simulink library "MAN_Library"  (R2023a)
settings: Solver=ode45  StartTime=0.0  StopTime=10.0  RelTol=1e-3  EnableMultiTasking=on
undefined symbols (not defined in the file): EventID
libraries: $bdroot x33, simulink_need_slupdate x1
(part 1 of 2)
settings Model: Creator=u23d01  LastModifiedBy=u29w13
settings SolverCC: AlgebraicLoopSolver=TrustRegion
settings DataIOCC: LimitDataPoints=on  SaveFormat=Array  ReturnWorkspaceOutputs=off
settings OptimizationCC: LifeSpan=inf
settings DebuggingCC: UnderspecifiedInitializationDetection=Classic  MergeDetectMultiDrivingBlocksExec=none  SolverPrmCheckMsg=warning  UnconnectedInputMsg=warning  UnconnectedOutputMsg=warning  UnconnectedLineMsg=warning  AllowSymbolicDim=off  SFUnexpectedBacktrackingDiag=warning  SFNoUnconditionalDefaultTransitionDiag=warning  SFExecutionAtInitializationDiag=none  ArithmeticOperatorsInVariantConditions=warning
settings HardwareCC: ProdBitPerPointer=32  ProdBitPerSizeT=32  ProdBitPerPtrDiffT=32  ProdLargestAtomicFloat=None  ProdIntDivRoundTo=Undefined  ProdEndianess=Unspecified  ProdWordSize=32  ProdHWDeviceType=32-bit Generic
settings ModelReferenceCC: EnableRefExpFcnMdlSchedulingChecks=on  PropagateSignalLabelsOutOfModel=off
settings SFSimCC: SimUseLocalCustomCode=off  CustomCodeUndefinedFunction=UseInterfaceOnly
settings RTWCC: RTWUseLocalCustomCode=off
settings CodeAppCC: StateflowObjectComments=on
settings GRTTargetCC: TargetLangStandard=C89/C90 (ANSI)
settings ConfigComp: CovMetricSettings=dw  CovSaveCumulativeToWorkspaceVar=on  CovSaveSingleToWorkspaceVar=on  CovExternalEMLEnable=off

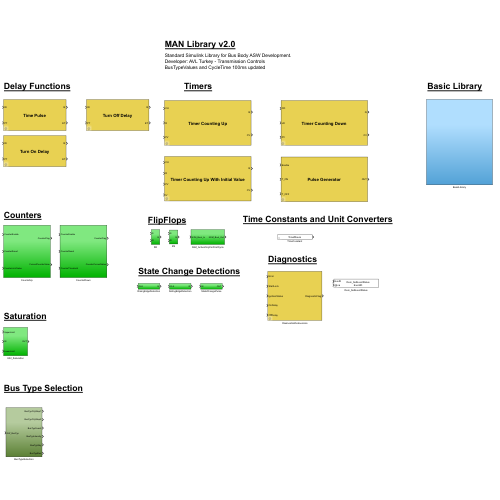
[thumbnail: Simulink's stored preview of the top-level diagram]
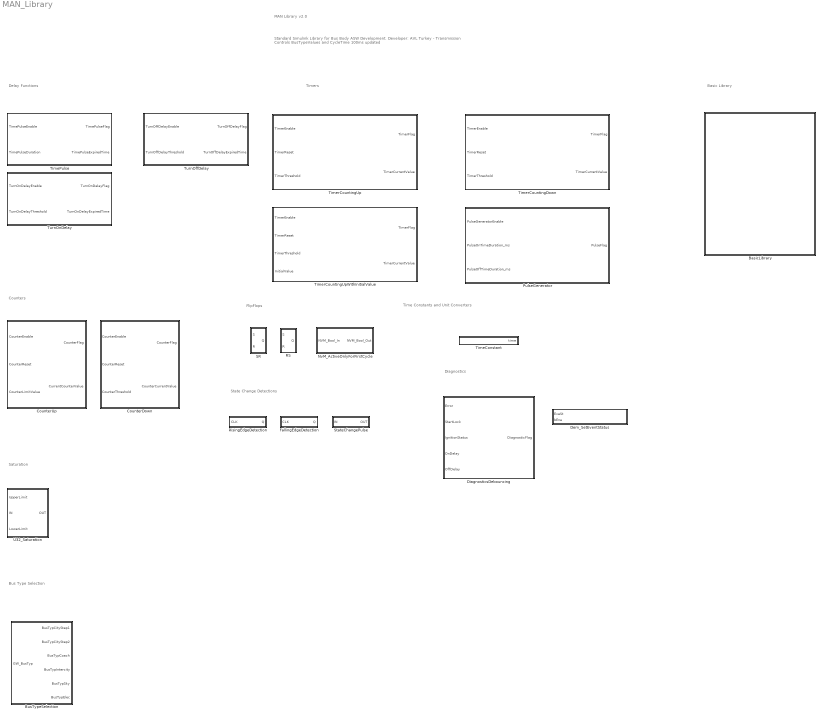
== system MAN_Library ==
  note: Standard Simulink Library for Bus Body ASW Development.
      | Developer: AVL Turkey - Transmission Controls
      | BusTypeValues and CycleTime 100ms updated
  note: Counters
  note: FlipFlops
  note: Saturation
  note: MAN Library v2.0
  note: Diagnostics
  note: Time Constants and Unit Converters
  note: State Change Detections
  note: Delay Functions
  note: Timers
  note: Basic Library
  note: Bus Type Selection
  BasicLibrary : Subsystem
  BusTypeSelection : Subsystem
  CounterDown : Subsystem
  CounterUp : Subsystem
  Dem_SetEventStatus : Subsystem  mask(AVL SL Blockset Dem_SetEventStatus){EventID=, SLB_DEMEventID=EventID}
      mask prompts: EventID "Dem Event ID legacy"; SLB_DEMEventID "DEM Event ID"
      mask help:
      | Interface block to call Dem_SetEventStatus.
      | The output of the block can be captured by using Dem_SetEventStatus blocks with the same EventID.
      mask init:
      | if strcmp(get(gcbh,'LinkStatus'),'resolved')
      |     % Enable mask
      |     set(gcbh,'MaskEnables',repmat({'on'},size(get(gcbh,'Maskenables'))))
      |     
      |     % Call block
      |     blk = SLBlockset.Blocks.Dem_SetEventStatus.Dem_SetEventStatus(gcbh);
      |     blk.initBlock();
      | else
      |     % Disable mask
      |     set(gcbh,'MaskEnables',repmat({'off'},size(get(gcbh,'Maskenables'))))
      | end
      mask DialogControl Control2 Prompt: Select
      mask DialogControl Control2 Callback: SLBlockset.Blocks.Dem_SetEventStatus.Dem_SetEventStatus.cb_selectVariable(gcbh,'Simulink.Parameter','SLB_DEMEventID');
      mask Display:
      | id = get_param(gcb,'SLB_DEMEventID');
      | text(0.55,0.9,sprintf('Dem_SetEventStatus\n%s', id),...
      |     'horizontalAlignment','center',...
      |     'verticalAlignment', 'top');
      | 
      | 
      | port_label('input',1,'EveSt');
      | port_label('input',2,'bEna');
  DiagnosticsDebouncing : Subsystem  mask(Diagnostics Debouncing){CycleTime=Cycle Time: 10 Ms}
      mask prompts: CycleTime "Select the Cycle Time:"
      mask TypeOptions CycleTime: Cycle Time: 1 Ms | Cycle Time: 10 Ms | Cycle Time: 100 Ms | Cycle Time: 1000 Ms
      mask Display:
      | %fprintf('PulseGenerator');
      | 
      | port_label('input', 1,'Error');
      | port_label('input', 2,'StartLock');
      | port_label('input', 3,'IgnitionStatus');
      | port_label('input', 4,'OnDelay');
      | port_label('input', 5,'OffDelay');
      | port_label('output',1,'DiagnosticFlag');
  FallingEdgeDetection : Subsystem
  NvM_ActiveOnlyForFirstCycle : Subsystem
  PulseGenerator : Subsystem  mask(Pulse Generator){CycleTime=Cycle Time: 10 Ms}
      mask prompts: CycleTime "Select the Cycle Time:"
      mask help:
      | Enable : Pulse generator enable
      | T_ON   : On time duration of the pulse
      | T_OFF  : Off time duration of the pulse
      | OUT    : Pulse flag
      mask TypeOptions CycleTime: Cycle Time: 1 Ms | Cycle Time: 10 Ms | Cycle Time: 100 Ms | Cycle Time: 1000 Ms
      mask Display:
      | disp('{\bf\fontsize{18}Pulse Generator}', 'texmode','on');
      | 
      | port_label('input', 1,'Enable');
      | port_label('input', 2,'T_ON');
      | port_label('input', 3,'T_OFF');
      | port_label('output',1,'OUT');
  RS : Subsystem
  RisingEdgeDetection : Subsystem
  SR : Subsystem
  StateChangePulse : Subsystem
  TimeConstant : Subsystem  mask{hours=0, minutes=0, seconds=0, miliseconds=0}
      mask prompts: hours "Hour"
      mask DialogControl TimeConstant Prompt: Time Constant
      mask Display:
      | timeDraw = 'Time#';
      | if( hours == 0 && minutes == 0 && seconds == 0 && miliseconds == 0)
      |     timeDraw = strcat(timeDraw,'0secs'),
      | else
      |     if( hours ~= 0)
      |         timeDraw = strcat(timeDraw,num2str(hours),'hours');
      |     end
      |     if( minutes ~= 0)
      |         timeDraw = strcat(timeDraw,num2str(minutes),'min');
      |     end
      |     if( seconds ~= 0)
      |         timeDraw = strcat(timeDraw,num2str(seconds),'sec');
      |     end
      |     if( miliseconds ~= 0)
      |         timeDraw = strcat(timeDraw,num2str(miliseconds),'ms');
      |     end
      | end
      | fprintf(timeDraw);
  TimePulse : Subsystem  mask(Time Pulse){CycleTime=Cycle Time: 10 Ms}
      mask prompts: CycleTime "Select the Cycle Time:"
      mask help:
      | This is a PULSE GENERATOR producing a pulse, if there is a positive-going edge at input IN. The length of the pulse which should be generated is defined by input PT. After the occurrence of the positive edge output Q is set to HIGH for the period of time defined in PT. Output ET counts the time - beginning with the occurrence of the positive edge - until the value set at PT has been reached. The value in ET is kept as long as the input IN has the state of HIGH.
      |
      | IN : Timer starting bit
      | PT : Preset time of timer
      | Q  : Time pulse flag
      | ET : Current value of timer
      mask TypeOptions CycleTime: Cycle Time: 1 Ms | Cycle Time: 10 Ms | Cycle Time: 100 Ms | Cycle Time: 1000 Ms
      mask Display:
      | disp('{\bf\fontsize{18}Time Pulse}', 'texmode','on');
      | 
      | port_label('input', 1,'IN');
      | port_label('input', 2,'PT');
      | port_label('output',1,'Q');
      | port_label('output',2,'ET');
  TimerCountingDown : Subsystem  mask(Timer Counting Down){CycleTime=Cycle Time: 10 Ms}
      mask prompts: CycleTime "Select the Cycle Time:"
      mask help:
      | This is a DOWN-COUNTER. The counter value can be set to the input value PV by input LD. An edge at input CD decrements the value by 1. The Boolean output Q is set on TRUE when the counter value reaches or falls below 0. The current counter value of the block can always be read from output CV.
      |
      | CD : Count down enable
      | LD : Load input
      | PV : Counter limit
      | Q  : Timer flag
      | CV : Current counter value
      mask TypeOptions CycleTime: Cycle Time: 1 Ms | Cycle Time: 10 Ms | Cycle Time: 100 Ms | Cycle Time: 1000 Ms
      mask Display:
      | disp('{\bf\fontsize{18}Timer Counting Down}', 'texmode','on');
      | 
      | port_label('input', 1,'CD');
      | port_label('input', 2,'LD');
      | port_label('input', 3,'PV');
      | port_label('output',1,'Q');
      | port_label('output',2,'CV');
  TimerCountingUp : Subsystem  mask(Timer Counting Up){CycleTime=Cycle Time: 10 Ms}
      mask prompts: CycleTime "Select the Cycle Time:"
      mask help:
      | This is an UP-COUNTER. The counter can be reset to 0 by the input R. An edge at input CU increments the value by 1. The input PV marks a limit at which the Boolean output Q is set on TRUE if the limit is reached or exceeded. The current counter value of the block can always be read from output CV.
      |
      | CU : Count up enable
      | R  : Timer Reset
      | PV : Counter limit
      | Q  : Timer flag
      | CV : Current counter value
      mask TypeOptions CycleTime: Cycle Time: 1 Ms | Cycle Time: 10 Ms | Cycle Time: 100 Ms | Cycle Time: 1000 Ms
      mask Display:
      | disp('{\bf\fontsize{18}Timer Counting Up}', 'texmode','on');
      | 
      | port_label('input', 1,'CU');
      | port_label('input', 2,'R');
      | port_label('input', 3,'PV');
      | port_label('output',1,'Q');
      | port_label('output',2,'CV');
      | 
      | 
      | % PortName_Button = get_param(gcb,'Buttons')
      | % if (PortName_Button == 'Cycle Time: 1 Ms')
      | %     CycleTime = uint32(1);
      | % elseif (PortName_Button == 'Cycle Time: 10 Ms')
      | %     CycleTime = uint32(10);
      | % elseif (PortName_Button == 'Cycle Time: 100 Ms')
      | %     CycleTime = uint32(100);
      | % else
      | %     CycleTime = uint32(1000);
      | % end
      | %
  TimerCountingUpWithInitialValue : Subsystem  mask(Timer Counting Up With Initial Value){CycleTime=Cycle Time: 10 Ms}
      mask prompts: CycleTime "Select the Cycle Time:"
      mask help:
      | This is an UP-COUNTER. The counter can be reset to 0 by the input R. An edge at input CU increments the value by 1 from starting initial value(IV). The input PV marks a limit at which the Boolean output Q is set on TRUE if the limit is reached or exceeded. The current counter value of the block can always be read from output CV.
      |
      | CU : Count up enable
      | R  : Timer Reset
      | PV : Counter limit
      | IV : Initial value
      | Q  : Timer flag
      | CV : Current counter value
      mask TypeOptions CycleTime: Cycle Time: 1 Ms | Cycle Time: 10 Ms | Cycle Time: 100 Ms | Cycle Time: 1000 Ms
      mask Display:
      | disp('{\bf\fontsize{18}Timer Counting Up With Initial Value}', 'texmode','on');
      | 
      | port_label('input', 1,'CU');
      | port_label('input', 2,'R');
      | port_label('input', 3,'PV');
      | port_label('input', 4,'IV');
      | port_label('output',1,'Q');
      | port_label('output',2,'CV');
  TurnOffDelay : Subsystem  mask(Turn Off Delay){CycleTime=Cycle Time: 10 Ms}
      mask prompts: CycleTime "Select the Cycle Time:"
      mask help:
      | This is an EDGE DELAY where the turning-off edge is delayed. The delay period is entered at input PT. The output Q is reset after turning off input IN, only after the delay period is over. Output ET counts the time - beginning with the occurrence of the negative edge - until the value set at PT has been reached. The output ET shows the expired time since turning input IN off until the input state of IN is put through to output Q.
      |
      | IN : Timer starting bit
      | PT : Preset time of timer
      | Q  : Time pulse flag
      | ET : Current value of timer
      mask TypeOptions CycleTime: Cycle Time: 1 Ms | Cycle Time: 10 Ms | Cycle Time: 100 Ms | Cycle Time: 1000 Ms
      mask Display:
      | disp('{\bf\fontsize{18}Turn Off Delay}', 'texmode','on');
      | 
      | port_label('input', 1,'IN');
      | port_label('input', 2,'PT');
      | port_label('output',1,'Q');
      | port_label('output',2,'ET');
  TurnOnDelay : Subsystem  mask(Turn On Delay){CycleTime=Cycle Time: 10 Ms}
      mask prompts: CycleTime "Select the Cycle Time:"
      mask help:
      | This is an EDGE DELAY where the turning-on edge is delayed. The delay period is entered at input PT. Output Q is set on TRUE after turning on input IN, only after the delay period is over. Output ET counts the time - beginning with the occurrence of the positive edge - until the value set at PT has been reached. The output ET shows the expired time since turning input IN on until the input state of IN is put through to output Q.
      |
      | IN : Timer starting bit
      | PT : Preset time of timer
      | Q  : Time up flag
      | ET : Current value of timer
      mask TypeOptions CycleTime: Cycle Time: 1 Ms | Cycle Time: 10 Ms | Cycle Time: 100 Ms | Cycle Time: 1000 Ms
      mask Display:
      | disp('{\bf\fontsize{18}Turn On Delay}', 'texmode','on');
      | 
      | port_label('input', 1,'IN');
      | port_label('input', 2,'PT');
      | port_label('output',1,'Q');
      | port_label('output',2,'ET');
  U32_Saturation : Subsystem

== system MAN_Library/BasicLibrary ==
  note: Delay Functions
  note: Timers
  note: Diagnostics
  DiagnosticsDebouncingOriginal : Subsystem
  PulseGeneratorOriginal : Subsystem
  TimePulseOriginal : Subsystem
  TimerCountingDownOriginal : Subsystem
  TimerCountingUpOriginal : Subsystem
  TimerCountingUpWithInitialValueOriginal : Subsystem
  TurnOffDelayOriginal : Subsystem
  TurnOnDelayOriginal : Subsystem

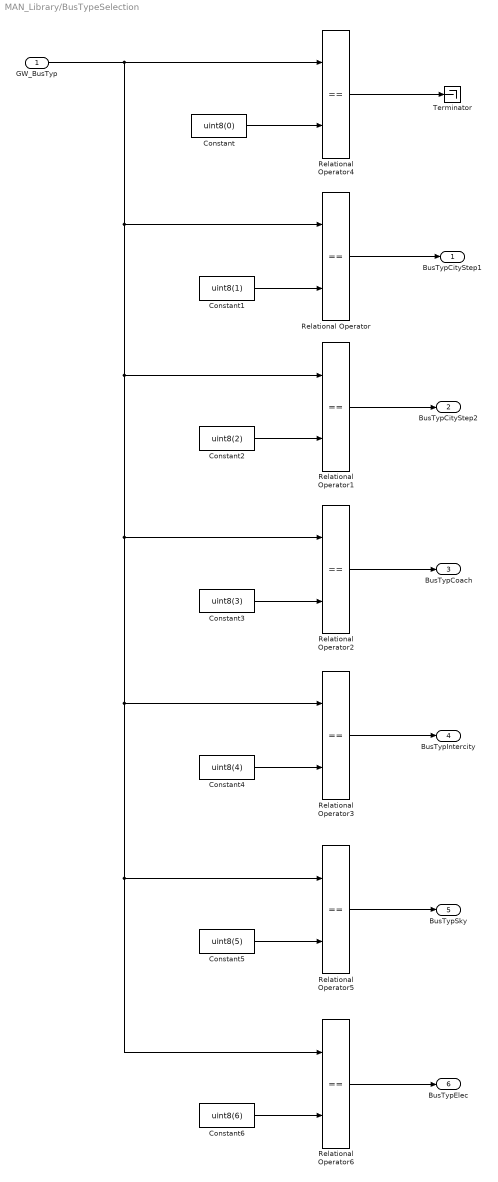
== system MAN_Library/BusTypeSelection ==
  GW_BusTyp : Inport
  Constant : Constant  Value=uint8(0)
  Constant1 : Constant  Value=uint8(1)
  Constant2 : Constant  Value=uint8(2)
  Constant3 : Constant  Value=uint8(3)
  Constant4 : Constant  Value=uint8(4)
  Constant5 : Constant  Value=uint8(5)
  Constant6 : Constant  Value=uint8(6)
  Relational Operator{,1..6} (7 alike) : RelationalOperator  Operator===  OutDataTypeStr=boolean  InputSameDT=off
  Terminator : Terminator
  BusTypCityStep1 : Outport
  BusTypCityStep2 : Outport  Port=2
  BusTypCoach : Outport  Port=3
  BusTypIntercity : Outport  Port=4
  BusTypSky : Outport  Port=5
  BusTypElec : Outport  Port=6
  wires:
  Constant2/1 -> Relational Operator1/2
  Constant3/1 -> Relational Operator2/2
  Relational Operator2/1 -> BusTypCoach/1
  Relational Operator1/1 -> BusTypCityStep2/1
  Relational Operator3/1 -> BusTypIntercity/1
  Relational Operator/1 -> BusTypCityStep1/1
  Constant1/1 -> Relational Operator/2
  Constant4/1 -> Relational Operator3/2
  Constant/1 -> Relational Operator4/2
  Relational Operator4/1 -> Terminator/1
  Relational Operator5/1 -> BusTypSky/1
  Constant5/1 -> Relational Operator5/2
  Constant6/1 -> Relational Operator6/2
  GW_BusTyp/1 -> Relational Operator4/1, Relational Operator6/1, Relational Operator5/1, Relational Operator3/1, Relational Operator2/1, Relational Operator1/1, Relational Operator/1
  Relational Operator6/1 -> BusTypElec/1

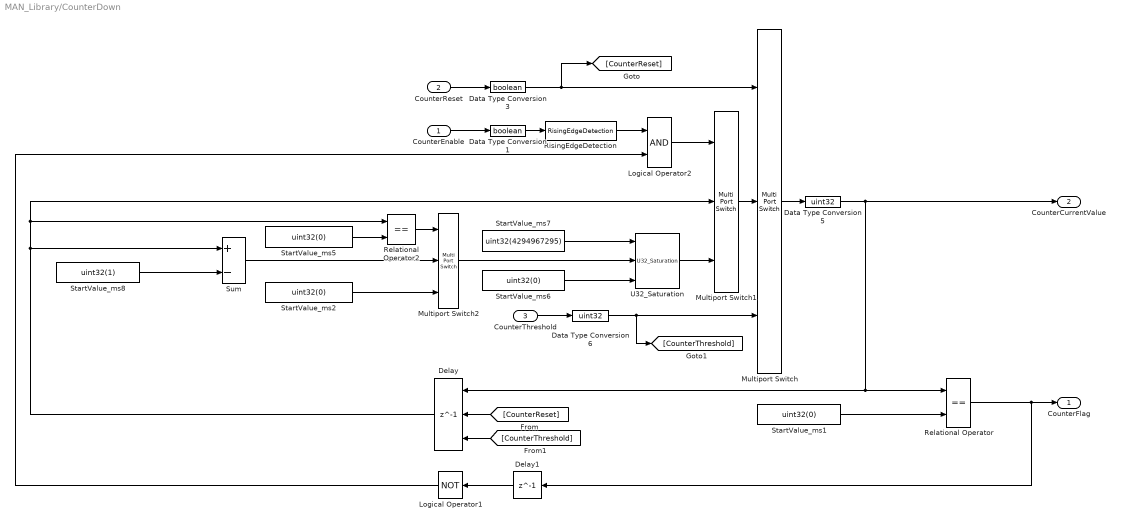
== system MAN_Library/CounterDown ==
  CounterEnable : Inport
  CounterReset : Inport  Port=2
  CounterThreshold : Inport  Port=3
  Data Type Conversion1 : DataTypeConversion  OutDataTypeStr=boolean  SaturateOnIntegerOverflow=off  RndMeth=Floor
  Data Type Conversion3 : DataTypeConversion  OutDataTypeStr=boolean  SaturateOnIntegerOverflow=off  RndMeth=Floor
  Data Type Conversion5 : DataTypeConversion  OutDataTypeStr=uint32  SaturateOnIntegerOverflow=off  RndMeth=Floor
  Data Type Conversion6 : DataTypeConversion  OutDataTypeStr=uint32  SaturateOnIntegerOverflow=off  RndMeth=Floor
  Delay : Delay  DelayLength=1  InitialConditionSource=Input port  InitialCondition=0  ExternalReset=Rising
      settings: InputPortMap=u0,r5,p4
  Delay1 : Delay  DelayLength=1  InitialCondition=0
  Logical Operator1 : Logic  Operator=NOT  AllPortsSameDT=off  OutDataTypeStr=boolean
  Logical Operator2 : Logic  AllPortsSameDT=off  OutDataTypeStr=boolean
  Multiport Switch : MultiPortSwitch  DataPortOrder=Zero-based contiguous  Inputs=2  zeroidx=on  SaturateOnIntegerOverflow=off  InputSameDT=off
  Multiport Switch1 : MultiPortSwitch  DataPortOrder=Zero-based contiguous  Inputs=2  zeroidx=on  SaturateOnIntegerOverflow=off  InputSameDT=off
  Multiport Switch2 : MultiPortSwitch  DataPortOrder=Zero-based contiguous  Inputs=2  zeroidx=on  SaturateOnIntegerOverflow=off  InputSameDT=off
  Relational Operator : RelationalOperator  Operator===  OutDataTypeStr=boolean  InputSameDT=off
  Relational Operator2 : RelationalOperator  Operator===  OutDataTypeStr=boolean  InputSameDT=off
  RisingEdgeDetection : $bdroot/RisingEdgeDetection  SystemSampleTime=-1  VariantActivationTime=update diagram  Latency=0  AutoFrameSizeCalculation=off
  StartValue_ms{1..2,5..6} (4 alike) : Constant  Value=uint32(0)  OutDataTypeStr=uint32
  StartValue_ms7 : Constant  Value=uint32(4294967295)  OutDataTypeStr=uint32
  StartValue_ms8 : Constant  Value=uint32(1)  OutDataTypeStr=uint32
  Sum : Sum  Inputs=+-
  U32_Saturation : $bdroot/U32_Saturation  SystemSampleTime=-1  VariantActivationTime=update diagram  Latency=0  AutoFrameSizeCalculation=off
  CounterFlag : Outport
  CounterCurrentValue : Outport  Port=2
  wires:
  [CounterReset] -> Delay/2
  CounterThreshold/1 -> Data Type Conversion6/1
  Multiport Switch1/1 -> Multiport Switch/2
  Relational Operator/1 -> Delay1/1, CounterFlag/1
  Multiport Switch/1 -> Data Type Conversion5/1
  Data Type Conversion1/1 -> RisingEdgeDetection/1
  Data Type Conversion5/1 -> Relational Operator/1, Delay/1, CounterCurrentValue/1
  Logical Operator2/1 -> Multiport Switch1/1
  Logical Operator1/1 -> Logical Operator2/2
  U32_Saturation/1 -> Multiport Switch1/3
  Delay1/1 -> Logical Operator1/1
  StartValue_ms7/1 -> U32_Saturation/1
  Delay/1 -> Sum/1, Relational Operator2/1, Multiport Switch1/2
  Relational Operator2/1 -> Multiport Switch2/1
  StartValue_ms2/1 -> Multiport Switch2/3
  Sum/1 -> Multiport Switch2/2
  Multiport Switch2/1 -> U32_Saturation/2
  StartValue_ms6/1 -> U32_Saturation/3
  StartValue_ms8/1 -> Sum/2
  StartValue_ms1/1 -> Relational Operator/2
  CounterEnable/1 -> Data Type Conversion1/1
  Data Type Conversion6/1 -> [CounterThreshold], Multiport Switch/3
  [CounterThreshold] -> Delay/3
  Data Type Conversion3/1 -> Multiport Switch/1, [CounterReset]
  CounterReset/1 -> Data Type Conversion3/1
  RisingEdgeDetection/1 -> Logical Operator2/1
  StartValue_ms5/1 -> Relational Operator2/2

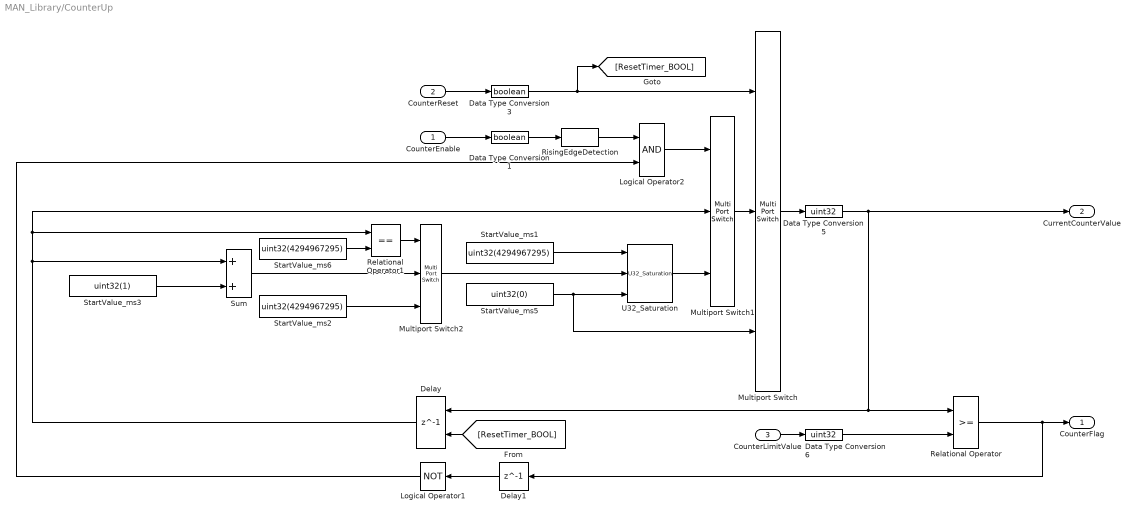
== system MAN_Library/CounterUp ==
  CounterEnable : Inport
  CounterReset : Inport  Port=2
  CounterLimitValue : Inport  Port=3
  Data Type Conversion1 : DataTypeConversion  OutDataTypeStr=boolean  SaturateOnIntegerOverflow=off  RndMeth=Floor
  Data Type Conversion3 : DataTypeConversion  OutDataTypeStr=boolean  SaturateOnIntegerOverflow=off  RndMeth=Floor
  Data Type Conversion5 : DataTypeConversion  OutDataTypeStr=uint32  SaturateOnIntegerOverflow=off  RndMeth=Floor
  Data Type Conversion6 : DataTypeConversion  OutDataTypeStr=uint32  SaturateOnIntegerOverflow=off  RndMeth=Floor
  Delay : Delay  DelayLength=1  InitialCondition=0  ExternalReset=Rising
      settings: InputPortMap=u0,r5
  Delay1 : Delay  DelayLength=1  InitialCondition=0
  Logical Operator1 : Logic  Operator=NOT  AllPortsSameDT=off  OutDataTypeStr=boolean
  Logical Operator2 : Logic  AllPortsSameDT=off  OutDataTypeStr=boolean
  Multiport Switch : MultiPortSwitch  DataPortOrder=Zero-based contiguous  Inputs=2  zeroidx=on  SaturateOnIntegerOverflow=off  InputSameDT=off
  Multiport Switch1 : MultiPortSwitch  DataPortOrder=Zero-based contiguous  Inputs=2  zeroidx=on  SaturateOnIntegerOverflow=off  InputSameDT=off
  Multiport Switch2 : MultiPortSwitch  DataPortOrder=Zero-based contiguous  Inputs=2  zeroidx=on  SaturateOnIntegerOverflow=off  InputSameDT=off
  Relational Operator : RelationalOperator  OutDataTypeStr=boolean  InputSameDT=off
  Relational Operator1 : RelationalOperator  Operator===  OutDataTypeStr=boolean  InputSameDT=off
  RisingEdgeDetection : $bdroot/RisingEdgeDetection  SystemSampleTime=-1  VariantActivationTime=update diagram  Latency=0  AutoFrameSizeCalculation=off
  StartValue_ms1 : Constant  Value=uint32(4294967295)  OutDataTypeStr=uint32
  StartValue_ms2 : Constant  Value=uint32(4294967295)  OutDataTypeStr=uint32
  StartValue_ms3 : Constant  Value=uint32(1)  OutDataTypeStr=uint32
  StartValue_ms5 : Constant  Value=uint32(0)  OutDataTypeStr=uint32
  StartValue_ms6 : Constant  Value=uint32(4294967295)  OutDataTypeStr=uint32
  Sum : Sum
  U32_Saturation : $bdroot/U32_Saturation  SystemSampleTime=-1  VariantActivationTime=update diagram  Latency=0  AutoFrameSizeCalculation=off
  CounterFlag : Outport
  CurrentCounterValue : Outport  Port=2
  wires:
  [ResetTimer_BOOL] -> Delay/2
  CounterLimitValue/1 -> Data Type Conversion6/1
  CounterEnable/1 -> Data Type Conversion1/1
  Multiport Switch1/1 -> Multiport Switch/2
  Relational Operator/1 -> Delay1/1, CounterFlag/1
  Multiport Switch/1 -> Data Type Conversion5/1
  RisingEdgeDetection/1 -> Logical Operator2/1
  Data Type Conversion5/1 -> Relational Operator/1, Delay/1, CurrentCounterValue/1
  Logical Operator2/1 -> Multiport Switch1/1
  Logical Operator1/1 -> Logical Operator2/2
  U32_Saturation/1 -> Multiport Switch1/3
  Delay1/1 -> Logical Operator1/1
  StartValue_ms1/1 -> U32_Saturation/1
  CounterReset/1 -> Data Type Conversion3/1
  Data Type Conversion3/1 -> [ResetTimer_BOOL], Multiport Switch/1
  StartValue_ms6/1 -> Relational Operator1/2
  Delay/1 -> Sum/1, Relational Operator1/1, Multiport Switch1/2
  Relational Operator1/1 -> Multiport Switch2/1
  StartValue_ms2/1 -> Multiport Switch2/3
  Sum/1 -> Multiport Switch2/2
  Multiport Switch2/1 -> U32_Saturation/2
  StartValue_ms5/1 -> Multiport Switch/3, U32_Saturation/3
  Data Type Conversion1/1 -> RisingEdgeDetection/1
  StartValue_ms3/1 -> Sum/2
  Data Type Conversion6/1 -> Relational Operator/2

== system MAN_Library/Dem_SetEventStatus ==
  EveSt : Inport
  bEna : Inport  Port=2
  DEM_EventID : Constant  Value=SLB_DEMEventID  SampleTime=-1
  Dem_SetEventStatus_Enable : Subsystem
  wires:
  DEM_EventID/1 -> Dem_SetEventStatus_Enable/1(EventID)
  EveSt/1 -> Dem_SetEventStatus_Enable/2(EveSt)
  bEna/1 -> Dem_SetEventStatus_Enable/Enable

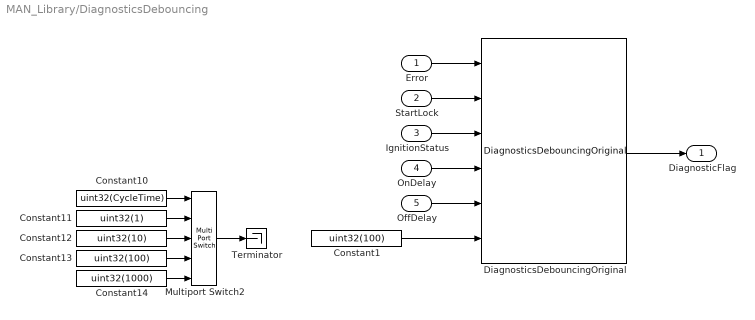
== system MAN_Library/DiagnosticsDebouncing ==
  Error : Inport
  StartLock : Inport  Port=2
  IgnitionStatus : Inport  Port=3
  OnDelay : Inport  Port=4
  OffDelay : Inport  Port=5
  Constant1 : Constant  Value=uint32(100)  OutDataTypeStr=uint32
  Constant10 : Constant  Value=uint32(CycleTime)  OutDataTypeStr=uint32
  Constant11 : Constant  Value=uint32(1)  OutDataTypeStr=uint32
  Constant12 : Constant  Value=uint32(10)  OutDataTypeStr=uint32
  Constant13 : Constant  Value=uint32(100)  OutDataTypeStr=uint32
  Constant14 : Constant  Value=uint32(1000)  OutDataTypeStr=uint32
  DiagnosticsDebouncingOriginal : $bdroot/BasicLibrary/DiagnosticsDebouncingOriginal  SystemSampleTime=-1  VariantActivationTime=update diagram  Latency=0  AutoFrameSizeCalculation=off
  Multiport Switch2 : MultiPortSwitch  Inputs=4  SaturateOnIntegerOverflow=off  InputSameDT=off
  Terminator : Terminator
  DiagnosticFlag : Outport
  wires:
  IgnitionStatus/1 -> DiagnosticsDebouncingOriginal/3
  OnDelay/1 -> DiagnosticsDebouncingOriginal/4
  StartLock/1 -> DiagnosticsDebouncingOriginal/2
  OffDelay/1 -> DiagnosticsDebouncingOriginal/5
  DiagnosticsDebouncingOriginal/1 -> DiagnosticFlag/1
  Error/1 -> DiagnosticsDebouncingOriginal/1
  Constant11/1 -> Multiport Switch2/2
  Constant12/1 -> Multiport Switch2/3
  Constant14/1 -> Multiport Switch2/5
  Constant13/1 -> Multiport Switch2/4
  Constant10/1 -> Multiport Switch2/1
  Multiport Switch2/1 -> Terminator/1
  Constant1/1 -> DiagnosticsDebouncingOriginal/6

== system MAN_Library/FallingEdgeDetection ==
  CLK : Inport
  Constant : Constant  Value=boolean(0)  OutDataTypeStr=boolean
  Data Type Conversion1 : DataTypeConversion  OutDataTypeStr=boolean  SaturateOnIntegerOverflow=off  RndMeth=Floor
  Logical Operator1 : Logic  AllPortsSameDT=off  OutDataTypeStr=boolean
  Relational Operator2 : RelationalOperator  Operator=~=  OutDataTypeStr=boolean  InputSameDT=off
  Relational Operator3 : RelationalOperator  Operator===  OutDataTypeStr=boolean  InputSameDT=off
  Unit Delay1 : UnitDelay  SampleTime=-1  HasFrameUpgradeWarning=on
  Q : Outport
  wires:
  Unit Delay1/1 -> Relational Operator2/1
  Relational Operator2/1 -> Logical Operator1/1
  Relational Operator3/1 -> Logical Operator1/2
  Logical Operator1/1 -> Q/1
  CLK/1 -> Data Type Conversion1/1
  Constant/1 -> Relational Operator3/2
  Data Type Conversion1/1 -> Relational Operator3/1, Relational Operator2/2, Unit Delay1/1

== system MAN_Library/NvM_ActiveOnlyForFirstCycle ==
  NVM_Bool_In : Inport
  Constant2 : Constant  Value=boolean(1)  OutDataTypeStr=boolean
  Constant3 : Constant  Value=boolean(0)  OutDataTypeStr=boolean
  Data Type Conversion2 : DataTypeConversion  OutDataTypeStr=boolean  SaturateOnIntegerOverflow=off  RndMeth=Floor
  Logical Operator : Logic  AllPortsSameDT=off  OutDataTypeStr=boolean
  Unit Delay External IC : simulink_need_slupdate/Unit Delay External IC  tsamp=-1
  NVM_Bool_Out : Outport
  wires:
  NVM_Bool_In/1 -> Data Type Conversion2/1
  Logical Operator/1 -> NVM_Bool_Out/1
  Unit Delay External IC/1 -> Logical Operator/2
  Constant3/1 -> Unit Delay External IC/1
  Constant2/1 -> Unit Delay External IC/2
  Data Type Conversion2/1 -> Logical Operator/1

== system MAN_Library/PulseGenerator ==
  PulseGeneratorEnable : Inport
  PulseOnTimeDuration_ms : Inport  Port=2
  PulseOffTimeDuration_ms : Inport  Port=3
  Constant1 : Constant  Value=uint32(100)  OutDataTypeStr=uint32
  Constant10 : Constant  Value=uint32(CycleTime)  OutDataTypeStr=uint32
  Constant11 : Constant  Value=uint32(1)  OutDataTypeStr=uint32
  Constant12 : Constant  Value=uint32(10)  OutDataTypeStr=uint32
  Constant13 : Constant  Value=uint32(100)  OutDataTypeStr=uint32
  Constant14 : Constant  Value=uint32(1000)  OutDataTypeStr=uint32
  Multiport Switch2 : MultiPortSwitch  Inputs=4  SaturateOnIntegerOverflow=off  InputSameDT=off
  PulseGeneratorOriginal : $bdroot/BasicLibrary/PulseGeneratorOriginal  SystemSampleTime=-1  VariantActivationTime=update diagram  Latency=0  AutoFrameSizeCalculation=off
  Terminator : Terminator
  PulseFlag : Outport
  wires:
  PulseGeneratorEnable/1 -> PulseGeneratorOriginal/1
  PulseOnTimeDuration_ms/1 -> PulseGeneratorOriginal/2
  PulseOffTimeDuration_ms/1 -> PulseGeneratorOriginal/3
  PulseGeneratorOriginal/1 -> PulseFlag/1
  Constant11/1 -> Multiport Switch2/2
  Constant12/1 -> Multiport Switch2/3
  Constant14/1 -> Multiport Switch2/5
  Constant13/1 -> Multiport Switch2/4
  Constant10/1 -> Multiport Switch2/1
  Multiport Switch2/1 -> Terminator/1
  Constant1/1 -> PulseGeneratorOriginal/4

== system MAN_Library/RS ==
  S : Inport
  R : Inport  Port=2
  Constant2 : Constant  Value=boolean(1)  OutDataTypeStr=boolean
  Constant3 : Constant  Value=boolean(0)  OutDataTypeStr=boolean
  Data Type Conversion1 : DataTypeConversion  OutDataTypeStr=boolean  SaturateOnIntegerOverflow=off  RndMeth=Floor
  Data Type Conversion2 : DataTypeConversion  OutDataTypeStr=boolean  SaturateOnIntegerOverflow=off  RndMeth=Floor
  Multiport Switch : MultiPortSwitch  DataPortOrder=Zero-based contiguous  Inputs=2  zeroidx=on  SaturateOnIntegerOverflow=off  InputSameDT=off
  Multiport Switch2 : MultiPortSwitch  DataPortOrder=Zero-based contiguous  Inputs=2  zeroidx=on  SaturateOnIntegerOverflow=off  InputSameDT=off
  Unit Delay : UnitDelay  SampleTime=-1  HasFrameUpgradeWarning=on
  Q : Outport
  wires:
  S/1 -> Data Type Conversion2/1
  Constant2/1 -> Multiport Switch/3
  Unit Delay/1 -> Multiport Switch/2
  R/1 -> Data Type Conversion1/1
  Constant3/1 -> Multiport Switch2/3
  Multiport Switch/1 -> Multiport Switch2/2
  Multiport Switch2/1 -> Q/1, Unit Delay/1
  Data Type Conversion2/1 -> Multiport Switch/1
  Data Type Conversion1/1 -> Multiport Switch2/1

== system MAN_Library/RisingEdgeDetection ==
  CLK : Inport
  Constant : Constant  Value=boolean(1)  OutDataTypeStr=boolean
  Data Type Conversion1 : DataTypeConversion  OutDataTypeStr=boolean  SaturateOnIntegerOverflow=off  RndMeth=Floor
  Logical Operator : Logic  AllPortsSameDT=off  OutDataTypeStr=boolean
  Relational Operator : RelationalOperator  Operator=~=  OutDataTypeStr=boolean  InputSameDT=off
  Relational Operator1 : RelationalOperator  Operator===  OutDataTypeStr=boolean  InputSameDT=off
  Unit Delay : UnitDelay  SampleTime=-1  HasFrameUpgradeWarning=on
  Q : Outport
  wires:
  CLK/1 -> Data Type Conversion1/1
  Unit Delay/1 -> Relational Operator/1
  Relational Operator/1 -> Logical Operator/1
  Relational Operator1/1 -> Logical Operator/2
  Logical Operator/1 -> Q/1
  Constant/1 -> Relational Operator1/2
  Data Type Conversion1/1 -> Unit Delay/1, Relational Operator/2, Relational Operator1/1

== system MAN_Library/SR ==
  S : Inport
  R : Inport  Port=2
  Constant1 : Constant  Value=boolean(1)  OutDataTypeStr=boolean
  Constant3 : Constant  Value=boolean(0)  OutDataTypeStr=boolean
  Data Type Conversion1 : DataTypeConversion  OutDataTypeStr=boolean  SaturateOnIntegerOverflow=off  RndMeth=Floor
  Data Type Conversion2 : DataTypeConversion  OutDataTypeStr=boolean  SaturateOnIntegerOverflow=off  RndMeth=Floor
  Multiport Switch : MultiPortSwitch  DataPortOrder=Zero-based contiguous  Inputs=2  zeroidx=on  SaturateOnIntegerOverflow=off  InputSameDT=off
  Multiport Switch1 : MultiPortSwitch  DataPortOrder=Zero-based contiguous  Inputs=2  zeroidx=on  SaturateOnIntegerOverflow=off  InputSameDT=off
  Unit Delay : UnitDelay  SampleTime=-1  HasFrameUpgradeWarning=on
  Q : Outport
  wires:
  S/1 -> Data Type Conversion2/1
  Constant1/1 -> Multiport Switch/3
  Multiport Switch1/1 -> Multiport Switch/2
  R/1 -> Data Type Conversion1/1
  Unit Delay/1 -> Multiport Switch1/2
  Multiport Switch/1 -> Q/1, Unit Delay/1
  Constant3/1 -> Multiport Switch1/3
  Data Type Conversion1/1 -> Multiport Switch1/1
  Data Type Conversion2/1 -> Multiport Switch/1

== system MAN_Library/StateChangePulse ==
  note: This function replaces '2k+1 XOR' block to detect changes.
  IN : Inport
  Data Type Conversion1 : DataTypeConversion  OutDataTypeStr=boolean  SaturateOnIntegerOverflow=off  RndMeth=Floor
  Data Type Conversion2 : DataTypeConversion  Commented=on  OutDataTypeStr=boolean  SaturateOnIntegerOverflow=off  RndMeth=Floor
  Ground : Ground  Commented=on
  Logical Operator17 : Logic  Operator=XOR  AllPortsSameDT=off  OutDataTypeStr=boolean
  Relational Operator : RelationalOperator  Commented=on  Operator=~=  OutDataTypeStr=boolean  InputSameDT=off
  Terminator : Terminator  Commented=on
  Unit Delay : UnitDelay  SampleTime=-1  HasFrameUpgradeWarning=on
  Unit Delay1 : UnitDelay  Commented=on  SampleTime=-1  HasFrameUpgradeWarning=on
  OUT : Outport
  wires:
  Logical Operator17/1 -> OUT/1, Unit Delay/1
  Unit Delay/1 -> Logical Operator17/2
  Data Type Conversion1/1 -> Logical Operator17/1
  Data Type Conversion2/1 -> Relational Operator/2, Unit Delay1/1
  Relational Operator/1 -> Terminator/1
  Ground/1 -> Data Type Conversion2/1
  IN/1 -> Data Type Conversion1/1
  Unit Delay1/1 -> Relational Operator/1

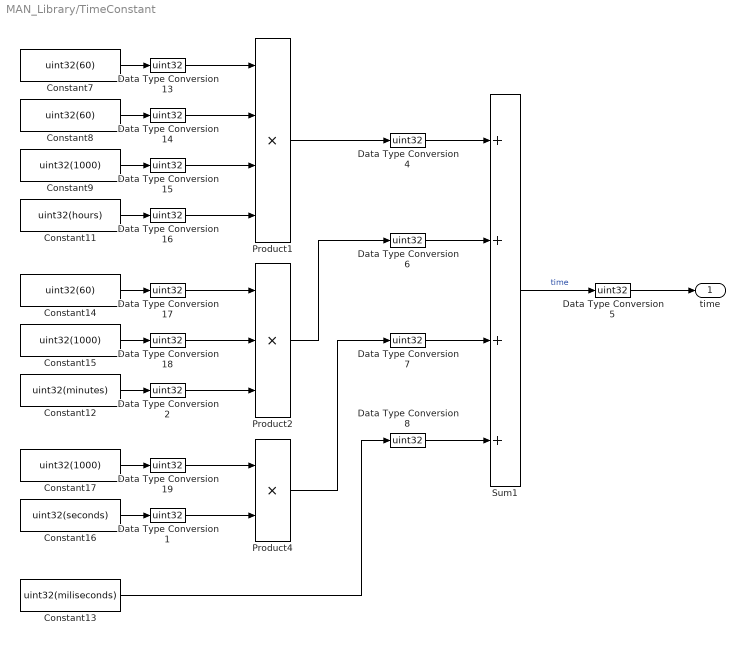
== system MAN_Library/TimeConstant ==
  Constant11 : Constant  Value=uint32(hours)  OutDataTypeStr=uint32
  Constant12 : Constant  Value=uint32(minutes)  OutDataTypeStr=uint32
  Constant13 : Constant  Value=uint32(miliseconds)  OutDataTypeStr=uint32
  Constant14 : Constant  Value=uint32(60)  OutDataTypeStr=uint32
  Constant15 : Constant  Value=uint32(1000)  OutDataTypeStr=uint32
  Constant16 : Constant  Value=uint32(seconds)  OutDataTypeStr=uint32
  Constant17 : Constant  Value=uint32(1000)  OutDataTypeStr=uint32
  Constant7 : Constant  Value=uint32(60)  OutDataTypeStr=uint32
  Constant8 : Constant  Value=uint32(60)  OutDataTypeStr=uint32
  Constant9 : Constant  Value=uint32(1000)  OutDataTypeStr=uint32
  Data Type Conversion{1..2,4..8,13..19} (14 alike) : DataTypeConversion  OutDataTypeStr=uint32  SaturateOnIntegerOverflow=off  RndMeth=Floor
  Product1 : Product  Inputs=4  OutDataTypeStr=uint32
  Product2 : Product  Inputs=3  OutDataTypeStr=uint32
  Product4 : Product  OutDataTypeStr=uint32
  Sum1 : Sum  Inputs=++++  AccumDataTypeStr=uint32
  time : Outport
  wires:
  Sum1/1 -> Data Type Conversion5/1  "time"
  Data Type Conversion5/1 -> time/1
  Constant7/1 -> Data Type Conversion13/1
  Data Type Conversion13/1 -> Product1/1
  Constant8/1 -> Data Type Conversion14/1
  Data Type Conversion14/1 -> Product1/2
  Constant9/1 -> Data Type Conversion15/1
  Data Type Conversion15/1 -> Product1/3
  Constant11/1 -> Data Type Conversion16/1
  Data Type Conversion16/1 -> Product1/4
  Constant12/1 -> Data Type Conversion2/1
  Constant14/1 -> Data Type Conversion17/1
  Data Type Conversion17/1 -> Product2/1
  Constant15/1 -> Data Type Conversion18/1
  Data Type Conversion18/1 -> Product2/2
  Constant17/1 -> Data Type Conversion19/1
  Data Type Conversion19/1 -> Product4/1
  Constant16/1 -> Data Type Conversion1/1
  Product1/1 -> Data Type Conversion4/1
  Product2/1 -> Data Type Conversion6/1
  Product4/1 -> Data Type Conversion7/1
  Data Type Conversion1/1 -> Product4/2
  Data Type Conversion2/1 -> Product2/3
  Constant13/1 -> Data Type Conversion8/1
  Data Type Conversion4/1 -> Sum1/1
  Data Type Conversion6/1 -> Sum1/2
  Data Type Conversion7/1 -> Sum1/3
  Data Type Conversion8/1 -> Sum1/4

== system MAN_Library/TimePulse ==
  TimePulseEnable : Inport
  TimePulseDuration : Inport  Port=2
  Constant1 : Constant  Value=uint32(100)  OutDataTypeStr=uint32
  Constant10 : Constant  Value=uint32(CycleTime)  OutDataTypeStr=uint32
  Constant11 : Constant  Value=uint32(1)  OutDataTypeStr=uint32
  Constant12 : Constant  Value=uint32(10)  OutDataTypeStr=uint32
  Constant13 : Constant  Value=uint32(100)  OutDataTypeStr=uint32
  Constant14 : Constant  Value=uint32(1000)  OutDataTypeStr=uint32
  Multiport Switch2 : MultiPortSwitch  Inputs=4  SaturateOnIntegerOverflow=off  InputSameDT=off
  Terminator : Terminator
  TimePulseOriginal : $bdroot/BasicLibrary/TimePulseOriginal  SystemSampleTime=-1  VariantActivationTime=update diagram  Latency=0  AutoFrameSizeCalculation=off
  TimePulseFlag : Outport
  TimePulseExpiredTime : Outport  Port=2
  wires:
  TimePulseOriginal/2 -> TimePulseExpiredTime/1
  TimePulseOriginal/1 -> TimePulseFlag/1
  TimePulseEnable/1 -> TimePulseOriginal/1
  TimePulseDuration/1 -> TimePulseOriginal/2
  Constant11/1 -> Multiport Switch2/2
  Constant12/1 -> Multiport Switch2/3
  Constant14/1 -> Multiport Switch2/5
  Constant13/1 -> Multiport Switch2/4
  Constant10/1 -> Multiport Switch2/1
  Multiport Switch2/1 -> Terminator/1
  Constant1/1 -> TimePulseOriginal/3

== system MAN_Library/TimerCountingDown ==
  TimerEnable : Inport
  TimerReset : Inport  Port=2
  TimerThreshold : Inport  Port=3
  Constant1 : Constant  Value=uint32(100)  OutDataTypeStr=uint32
  Constant10 : Constant  Value=uint32(CycleTime)  OutDataTypeStr=uint32
  Constant11 : Constant  Value=uint32(1)  OutDataTypeStr=uint32
  Constant12 : Constant  Value=uint32(10)  OutDataTypeStr=uint32
  Constant13 : Constant  Value=uint32(100)  OutDataTypeStr=uint32
  Constant14 : Constant  Value=uint32(1000)  OutDataTypeStr=uint32
  Multiport Switch2 : MultiPortSwitch  Inputs=4  SaturateOnIntegerOverflow=off  InputSameDT=off
  Terminator : Terminator
  TimerCountingDownOriginal : $bdroot/BasicLibrary/TimerCountingDownOriginal  SystemSampleTime=-1  VariantActivationTime=update diagram  Latency=0  AutoFrameSizeCalculation=off
  TimerFlag : Outport
  TimerCurrentValue : Outport  Port=2
  wires:
  TimerReset/1 -> TimerCountingDownOriginal/2
  TimerThreshold/1 -> TimerCountingDownOriginal/3
  TimerCountingDownOriginal/1 -> TimerFlag/1
  TimerCountingDownOriginal/2 -> TimerCurrentValue/1
  TimerEnable/1 -> TimerCountingDownOriginal/1
  Constant11/1 -> Multiport Switch2/2
  Constant12/1 -> Multiport Switch2/3
  Constant14/1 -> Multiport Switch2/5
  Constant13/1 -> Multiport Switch2/4
  Constant10/1 -> Multiport Switch2/1
  Multiport Switch2/1 -> Terminator/1
  Constant1/1 -> TimerCountingDownOriginal/4

== system MAN_Library/TimerCountingUp ==
  TimerEnable : Inport
  TimerReset : Inport  Port=2
  TimerThreshold : Inport  Port=3
  Constant11 : Constant  Value=uint32(1)  OutDataTypeStr=uint32
  Constant12 : Constant  Value=uint32(10)  OutDataTypeStr=uint32
  Constant13 : Constant  Value=uint32(100)  OutDataTypeStr=uint32
  Constant14 : Constant  Value=uint32(1000)  OutDataTypeStr=uint32
  Constant5 : Constant  Value=uint32(100)  OutDataTypeStr=uint32
  Constant6 : Constant  Value=uint32(CycleTime)  OutDataTypeStr=uint32
  Multiport Switch2 : MultiPortSwitch  Inputs=4  SaturateOnIntegerOverflow=off  InputSameDT=off
  Terminator : Terminator
  TimerCountingUpOriginal : $bdroot/BasicLibrary/TimerCountingUpOriginal  SystemSampleTime=-1  VariantActivationTime=update diagram  Latency=0  AutoFrameSizeCalculation=off
  TimerFlag : Outport
  TimerCurrentValue : Outport  Port=2
  wires:
  TimerEnable/1 -> TimerCountingUpOriginal/1
  TimerReset/1 -> TimerCountingUpOriginal/2
  TimerThreshold/1 -> TimerCountingUpOriginal/3
  TimerCountingUpOriginal/1 -> TimerFlag/1
  TimerCountingUpOriginal/2 -> TimerCurrentValue/1
  Constant11/1 -> Multiport Switch2/2
  Constant12/1 -> Multiport Switch2/3
  Constant14/1 -> Multiport Switch2/5
  Constant13/1 -> Multiport Switch2/4
  Constant6/1 -> Multiport Switch2/1
  Multiport Switch2/1 -> Terminator/1
  Constant5/1 -> TimerCountingUpOriginal/4

== system MAN_Library/TimerCountingUpWithInitialValue ==
  TimerEnable : Inport
  TimerReset : Inport  Port=2
  TimerThreshold : Inport  Port=3
  InitialValue : Inport  Port=4
  Constant1 : Constant  Value=uint32(100)  OutDataTypeStr=uint32
  Constant10 : Constant  Value=uint32(CycleTime)  OutDataTypeStr=uint32
  Constant11 : Constant  Value=uint32(1)  OutDataTypeStr=uint32
  Constant12 : Constant  Value=uint32(10)  OutDataTypeStr=uint32
  Constant13 : Constant  Value=uint32(100)  OutDataTypeStr=uint32
  Constant14 : Constant  Value=uint32(1000)  OutDataTypeStr=uint32
  Multiport Switch2 : MultiPortSwitch  Inputs=4  SaturateOnIntegerOverflow=off  InputSameDT=off
  Terminator : Terminator
  TimerCountingUpWithInitialValueOriginal : $bdroot/BasicLibrary/TimerCountingUpWithInitialValueOriginal  SystemSampleTime=-1  VariantActivationTime=update diagram  Latency=0  AutoFrameSizeCalculation=off
  TimerFlag : Outport
  TimerCurrentValue : Outport  Port=2
  wires:
  TimerEnable/1 -> TimerCountingUpWithInitialValueOriginal/1
  TimerReset/1 -> TimerCountingUpWithInitialValueOriginal/2
  TimerThreshold/1 -> TimerCountingUpWithInitialValueOriginal/3
  TimerCountingUpWithInitialValueOriginal/1 -> TimerFlag/1
  TimerCountingUpWithInitialValueOriginal/2 -> TimerCurrentValue/1
  InitialValue/1 -> TimerCountingUpWithInitialValueOriginal/4
  Constant11/1 -> Multiport Switch2/2
  Constant12/1 -> Multiport Switch2/3
  Constant14/1 -> Multiport Switch2/5
  Constant13/1 -> Multiport Switch2/4
  Constant10/1 -> Multiport Switch2/1
  Multiport Switch2/1 -> Terminator/1
  Constant1/1 -> TimerCountingUpWithInitialValueOriginal/5

== system MAN_Library/TurnOffDelay ==
  TurnOffDelayEnable : Inport
  TurnOffDelayThreshold : Inport  Port=2
  Constant1 : Constant  Value=uint32(100)  OutDataTypeStr=uint32
  Constant10 : Constant  Value=uint32(CycleTime)  OutDataTypeStr=uint32
  Constant11 : Constant  Value=uint32(1)  OutDataTypeStr=uint32
  Constant12 : Constant  Value=uint32(10)  OutDataTypeStr=uint32
  Constant13 : Constant  Value=uint32(100)  OutDataTypeStr=uint32
  Constant14 : Constant  Value=uint32(1000)  OutDataTypeStr=uint32
  Multiport Switch2 : MultiPortSwitch  Inputs=4  SaturateOnIntegerOverflow=off  InputSameDT=off
  Terminator : Terminator
  TurnOffDelayOriginal : $bdroot/BasicLibrary/TurnOffDelayOriginal  SystemSampleTime=-1  VariantActivationTime=update diagram  Latency=0  AutoFrameSizeCalculation=off
  TurnOffDelayFlag : Outport
  TurnOffDelayExpiredTime : Outport  Port=2
  wires:
  TurnOffDelayOriginal/2 -> TurnOffDelayExpiredTime/1
  TurnOffDelayOriginal/1 -> TurnOffDelayFlag/1
  TurnOffDelayThreshold/1 -> TurnOffDelayOriginal/2
  TurnOffDelayEnable/1 -> TurnOffDelayOriginal/1
  Constant11/1 -> Multiport Switch2/2
  Constant12/1 -> Multiport Switch2/3
  Constant14/1 -> Multiport Switch2/5
  Constant13/1 -> Multiport Switch2/4
  Constant10/1 -> Multiport Switch2/1
  Multiport Switch2/1 -> Terminator/1
  Constant1/1 -> TurnOffDelayOriginal/3

== system MAN_Library/TurnOnDelay ==
  TurnOnDelayEnable : Inport
  TurnOnDelayThreshold : Inport  Port=2
  Constant1 : Constant  Value=uint32(100)  OutDataTypeStr=uint32
  Constant11 : Constant  Value=uint32(1)  OutDataTypeStr=uint32
  Constant12 : Constant  Value=uint32(10)  OutDataTypeStr=uint32
  Constant13 : Constant  Value=uint32(100)  OutDataTypeStr=uint32
  Constant14 : Constant  Value=uint32(1000)  OutDataTypeStr=uint32
  Constant2 : Constant  Value=uint32(CycleTime)  OutDataTypeStr=uint32
  Multiport Switch2 : MultiPortSwitch  Inputs=4  SaturateOnIntegerOverflow=off  InputSameDT=off
  Terminator : Terminator
  TurnOnDelayOriginal : $bdroot/BasicLibrary/TurnOnDelayOriginal  SystemSampleTime=-1  VariantActivationTime=update diagram  Latency=0  AutoFrameSizeCalculation=off
  TurnOnDelayFlag : Outport
  TurnOnDelayExpiredTime : Outport  Port=2
  wires:
  TurnOnDelayEnable/1 -> TurnOnDelayOriginal/1
  TurnOnDelayThreshold/1 -> TurnOnDelayOriginal/2
  TurnOnDelayOriginal/2 -> TurnOnDelayExpiredTime/1
  TurnOnDelayOriginal/1 -> TurnOnDelayFlag/1
  Constant11/1 -> Multiport Switch2/2
  Constant12/1 -> Multiport Switch2/3
  Constant14/1 -> Multiport Switch2/5
  Constant13/1 -> Multiport Switch2/4
  Constant2/1 -> Multiport Switch2/1
  Multiport Switch2/1 -> Terminator/1
  Constant1/1 -> TurnOnDelayOriginal/3

== system MAN_Library/U32_Saturation ==
  UpperLimit : Inport
  IN : Inport  Port=2
  LowerLimit : Inport  Port=3
  Data Type Conversion{1..4} (4 alike) : DataTypeConversion  OutDataTypeStr=uint32  SaturateOnIntegerOverflow=off  RndMeth=Floor
  MinMax : MinMax  Inputs=2  OutDataTypeStr=uint32
  MinMax1 : MinMax  Function=max  Inputs=2  OutDataTypeStr=uint32
  OUT : Outport
  wires:
  UpperLimit/1 -> Data Type Conversion1/1
  IN/1 -> Data Type Conversion2/1
  MinMax/1 -> MinMax1/2
  LowerLimit/1 -> Data Type Conversion4/1
  MinMax1/1 -> Data Type Conversion3/1
  Data Type Conversion4/1 -> MinMax1/1
  Data Type Conversion1/1 -> MinMax/2
  Data Type Conversion2/1 -> MinMax/1
  Data Type Conversion3/1 -> OUT/1

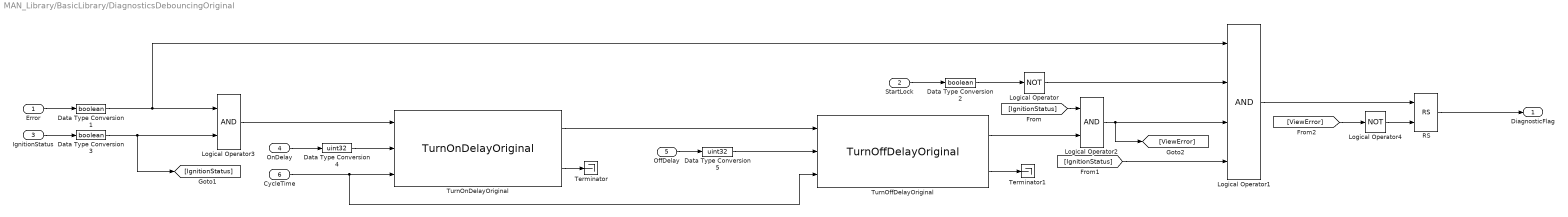
== system MAN_Library/BasicLibrary/DiagnosticsDebouncingOriginal ==
  Error : Inport
  StartLock : Inport  Port=2
  IgnitionStatus : Inport  Port=3
  OnDelay : Inport  Port=4
  OffDelay : Inport  Port=5
  CycleTime : Inport  Port=6
  Data Type Conversion1 : DataTypeConversion  OutDataTypeStr=boolean  SaturateOnIntegerOverflow=off  RndMeth=Floor
  Data Type Conversion2 : DataTypeConversion  OutDataTypeStr=boolean  SaturateOnIntegerOverflow=off  RndMeth=Floor
  Data Type Conversion3 : DataTypeConversion  OutDataTypeStr=boolean  SaturateOnIntegerOverflow=off  RndMeth=Floor
  Data Type Conversion4 : DataTypeConversion  OutDataTypeStr=uint32  SaturateOnIntegerOverflow=off  RndMeth=Floor
  Data Type Conversion5 : DataTypeConversion  OutDataTypeStr=uint32  SaturateOnIntegerOverflow=off  RndMeth=Floor
  Logical Operator : Logic  Operator=NOT  Inputs=1  AllPortsSameDT=off  OutDataTypeStr=boolean
  Logical Operator1 : Logic  Inputs=4  AllPortsSameDT=off  OutDataTypeStr=boolean
  Logical Operator2 : Logic  AllPortsSameDT=off  OutDataTypeStr=boolean
  Logical Operator3 : Logic  AllPortsSameDT=off  OutDataTypeStr=boolean
  Logical Operator4 : Logic  Operator=NOT  Inputs=1  AllPortsSameDT=off  OutDataTypeStr=boolean
  RS : $bdroot/RS  SystemSampleTime=-1  VariantActivationTime=update diagram  Latency=0  AutoFrameSizeCalculation=off
  Terminator : Terminator
  Terminator1 : Terminator
  "TurnOffDelayOriginal " : $bdroot/BasicLibrary/TurnOffDelayOriginal  SystemSampleTime=-1  VariantActivationTime=update diagram  Latency=0  AutoFrameSizeCalculation=off
  TurnOnDelayOriginal : $bdroot/BasicLibrary/TurnOnDelayOriginal  SystemSampleTime=-1  VariantActivationTime=update diagram  Latency=0  AutoFrameSizeCalculation=off
  DiagnosticFlag : Outport
  wires:
  OffDelay/1 -> Data Type Conversion5/1
  OnDelay/1 -> Data Type Conversion4/1
  IgnitionStatus/1 -> Data Type Conversion3/1
  StartLock/1 -> Data Type Conversion2/1
  Error/1 -> Data Type Conversion1/1
  Data Type Conversion3/1 -> [IgnitionStatus], Logical Operator3/2
  Logical Operator3/1 -> TurnOnDelayOriginal/1
  Data Type Conversion4/1 -> TurnOnDelayOriginal/2
  TurnOnDelayOriginal/1 -> "TurnOffDelayOriginal "/1
  TurnOnDelayOriginal/2 -> Terminator/1
  "TurnOffDelayOriginal "/2 -> Terminator1/1
  Data Type Conversion2/1 -> Logical Operator/1
  Logical Operator/1 -> Logical Operator1/2
  Data Type Conversion1/1 -> Logical Operator1/1, Logical Operator3/1
  [IgnitionStatus] -> Logical Operator2/1
  "TurnOffDelayOriginal "/1 -> Logical Operator2/2
  Logical Operator2/1 -> Logical Operator1/3, [ViewError]
  [IgnitionStatus] -> Logical Operator1/4
  Logical Operator1/1 -> RS/1
  Logical Operator4/1 -> RS/2
  [ViewError] -> Logical Operator4/1
  RS/1 -> DiagnosticFlag/1
  CycleTime/1 -> "TurnOffDelayOriginal "/3, TurnOnDelayOriginal/3
  Data Type Conversion5/1 -> "TurnOffDelayOriginal "/2

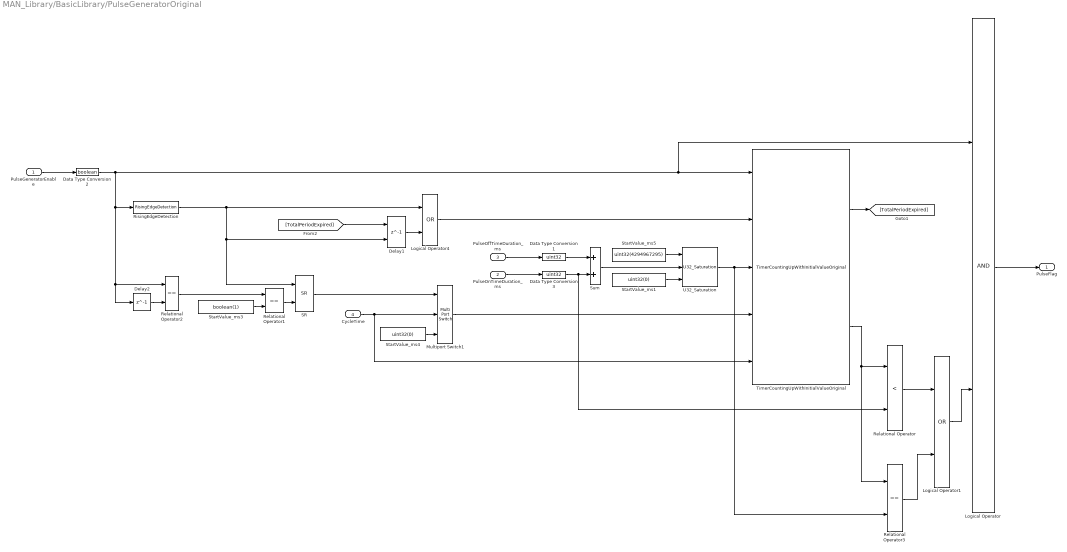
== system MAN_Library/BasicLibrary/PulseGeneratorOriginal ==
  PulseGeneratorEnable : Inport
  PulseOnTimeDuration_ms : Inport  Port=2
  PulseOffTimeDuration_ms : Inport  Port=3
  CycleTime : Inport  Port=4
  Data Type Conversion1 : DataTypeConversion  OutDataTypeStr=uint32  SaturateOnIntegerOverflow=off  RndMeth=Floor
  Data Type Conversion2 : DataTypeConversion  OutDataTypeStr=boolean  SaturateOnIntegerOverflow=off  RndMeth=Floor
  Data Type Conversion3 : DataTypeConversion  OutDataTypeStr=uint32  SaturateOnIntegerOverflow=off  RndMeth=Floor
  Delay1 : Delay  DelayLength=1  InitialCondition=0  ExternalReset=Rising
      settings: InputPortMap=u0,r5
  Delay2 : Delay  DelayLength=1  InitialCondition=0
  Logical Operator : Logic  AllPortsSameDT=off  OutDataTypeStr=boolean
  Logical Operator1 : Logic  Operator=OR  AllPortsSameDT=off  OutDataTypeStr=boolean
  Logical Operator4 : Logic  Operator=OR  AllPortsSameDT=off  OutDataTypeStr=boolean
  Multiport Switch1 : MultiPortSwitch  DataPortOrder=Zero-based contiguous  Inputs=2  zeroidx=on  SaturateOnIntegerOverflow=off  InputSameDT=off
  Relational Operator : RelationalOperator  Operator=<  OutDataTypeStr=boolean  InputSameDT=off
  Relational Operator1 : RelationalOperator  Operator===  OutDataTypeStr=boolean  InputSameDT=off
  Relational Operator2 : RelationalOperator  Operator===  OutDataTypeStr=boolean  InputSameDT=off
  Relational Operator3 : RelationalOperator  Operator===  OutDataTypeStr=boolean  InputSameDT=off
  RisingEdgeDetection : $bdroot/RisingEdgeDetection  SystemSampleTime=-1  VariantActivationTime=update diagram  Latency=0  AutoFrameSizeCalculation=off
  SR : $bdroot/SR  SystemSampleTime=-1  VariantActivationTime=update diagram  Latency=0  AutoFrameSizeCalculation=off
  StartValue_ms1 : Constant  Value=uint32(0)  OutDataTypeStr=uint32
  StartValue_ms3 : Constant  Value=boolean(1)  OutDataTypeStr=boolean
  StartValue_ms4 : Constant  Value=uint32(0)  OutDataTypeStr=uint32
  StartValue_ms5 : Constant  Value=uint32(4294967295)  OutDataTypeStr=uint32
  Sum : Sum
  TimerCountingUpWithInitialValueOriginal : $bdroot/BasicLibrary/TimerCountingUpWithInitialValueOriginal  SystemSampleTime=-1  VariantActivationTime=update diagram  Latency=0  AutoFrameSizeCalculation=off
  U32_Saturation : $bdroot/U32_Saturation  SystemSampleTime=-1  VariantActivationTime=update diagram  Latency=0  AutoFrameSizeCalculation=off
  PulseFlag : Outport
  wires:
  PulseGeneratorEnable/1 -> Data Type Conversion2/1
  Logical Operator/1 -> PulseFlag/1
  Data Type Conversion1/1 -> Sum/1
  StartValue_ms5/1 -> U32_Saturation/1
  StartValue_ms1/1 -> U32_Saturation/3
  Sum/1 -> U32_Saturation/2
  TimerCountingUpWithInitialValueOriginal/2 -> Relational Operator3/1, Relational Operator/1
  PulseOnTimeDuration_ms/1 -> Data Type Conversion3/1
  PulseOffTimeDuration_ms/1 -> Data Type Conversion1/1
  Relational Operator/1 -> Logical Operator1/1
  Logical Operator1/1 -> Logical Operator/2
  TimerCountingUpWithInitialValueOriginal/1 -> [TotalPeriodExpired]
  Data Type Conversion2/1 -> Delay2/1, Relational Operator2/1, RisingEdgeDetection/1, TimerCountingUpWithInitialValueOriginal/1, Logical Operator/1
  RisingEdgeDetection/1 -> SR/1, Delay1/2, Logical Operator4/1
  [TotalPeriodExpired] -> Delay1/1
  Delay1/1 -> Logical Operator4/2
  Logical Operator4/1 -> TimerCountingUpWithInitialValueOriginal/2
  U32_Saturation/1 -> TimerCountingUpWithInitialValueOriginal/3, Relational Operator3/2
  Multiport Switch1/1 -> TimerCountingUpWithInitialValueOriginal/4
  StartValue_ms4/1 -> Multiport Switch1/3
  SR/1 -> Multiport Switch1/1
  Relational Operator1/1 -> SR/2
  StartValue_ms3/1 -> Relational Operator1/2
  Relational Operator2/1 -> Relational Operator1/1
  Delay2/1 -> Relational Operator2/2
  Data Type Conversion3/1 -> Relational Operator/2, Sum/2
  Relational Operator3/1 -> Logical Operator1/2
  CycleTime/1 -> TimerCountingUpWithInitialValueOriginal/5, Multiport Switch1/2
